simulink model "Optimized_Quadrotor_Trajectory_PID_Control"  (R2021b)
settings: Solver=ode3  StartTime=0.0  StopTime=70  FixedStep=1e-3  RelTol=1e-3
libraries: vrlib x2
(part 1 of 2)
settings Model: Creator=hellb  LastModifiedBy=hellb
settings SolverCC: AlgebraicLoopSolver=TrustRegion
settings DataIOCC: ReturnWorkspaceOutputs=off
settings DebuggingCC: SFMachineParentedDataDiag=warning  ArithmeticOperatorsInVariantConditions=warning
settings SFSimCC: SimUseLocalCustomCode=off  CustomCodeUndefinedFunction=UseInterfaceOnly
settings RTWCC: RTWUseLocalCustomCode=off

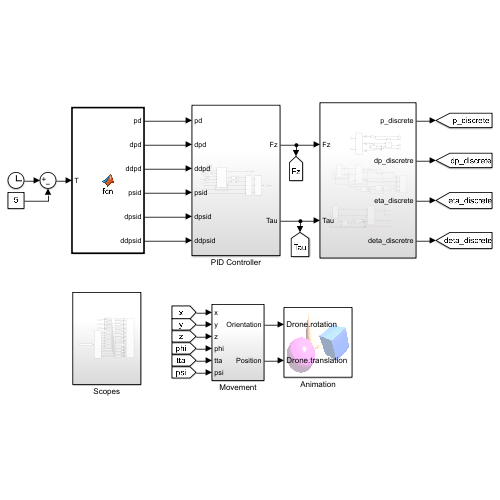
[thumbnail: Simulink's stored preview of the top-level diagram]
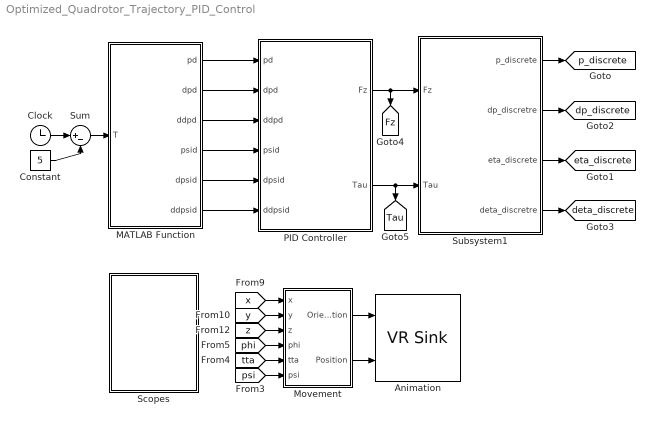
== system Optimized_Quadrotor_Trajectory_PID_Control ==
  Animation : vrlib/VR Sink  InstantiateOnLoad=on  SampleTime=0.01  ViewEnable=on  RemoteChange=off  RemoteView=off  FieldsWritten=Drone.rotation.4.1.1.double#Drone.translation.3.1.1.double  WorldFileName=Animation\hummingbird.wrl  AutoView=off  VideoDimensions=[]  AllowVariableSize=off
  Clock : Clock
  Constant : Constant  Value=5
  MATLAB Function : MATLAB Function  TreatAsAtomicUnit=on
  Movement : Subsystem
  PID Controller : Subsystem
  Scopes : Subsystem
  Subsystem1 : Subsystem
  Sum : Sum  Inputs=|+-
  tag scope: Fz=global, Tau=global, deta_discrete=global, dp_discrete=global, eta_discrete=global, p_discrete=global
  wires:
  [tta] -> Movement/5(tta)
  Movement/1(Orientation) -> Animation/1
  [z] -> Movement/3(z)
  Movement/2(Position) -> Animation/2
  [psi] -> Movement/6(psi)
  [y] -> Movement/2(y)
  [phi] -> Movement/4(phi)
  [x] -> Movement/1(x)
  Clock/1 -> Sum/1
  PID Controller/2(Tau) -> [Tau], Subsystem1/2(Tau)
  Subsystem1/1(p_discrete) -> [p_discrete]
  Subsystem1/3(eta_discrete) -> [eta_discrete]
  PID Controller/1(Fz) -> [Fz], Subsystem1/1(Fz)
  Subsystem1/2(dp_discretre) -> [dp_discrete]
  Subsystem1/4(deta_discretre) -> [deta_discrete]
  Sum/1 -> MATLAB Function/1(T)
  Constant/1 -> Sum/2
  MATLAB Function/1(pd) -> PID Controller/1(pd)
  MATLAB Function/2(dpd) -> PID Controller/2(dpd)
  MATLAB Function/3(ddpd) -> PID Controller/3(ddpd)
  MATLAB Function/4(psid) -> PID Controller/4(psid)
  MATLAB Function/5(dpsid) -> PID Controller/5(dpsid)
  MATLAB Function/6(ddpsid) -> PID Controller/6(ddpsid)

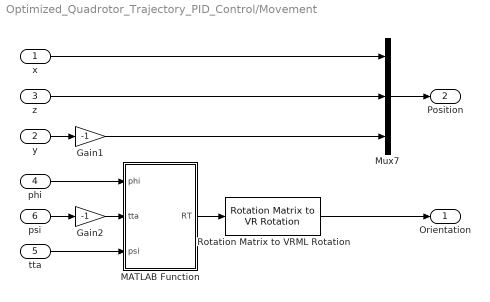
== system Optimized_Quadrotor_Trajectory_PID_Control/Movement ==
  x : Inport
  y : Inport  Port=2
  z : Inport  Port=3
  phi : Inport  Port=4
  tta : Inport  Port=5
  psi : Inport  Port=6
  Gain1 : Gain  Gain=-1
  Gain2 : Gain  Gain=-1
  MATLAB Function : MATLAB Function  TreatAsAtomicUnit=on
  Mux7 : Mux  Inputs=3
  Rotation Matrix to VRML Rotation : vrlib/Utilities/Rotation Matrix to VR Rotation  maxzero=1e-12
      settings: SourceProductBaseCode=SL
  Orientation : Outport  VectorParamsAs1DForOutWhenUnconnected=off
  Position : Outport  Port=2  VectorParamsAs1DForOutWhenUnconnected=off
  wires:
  Gain1/1 -> Mux7/3
  Rotation Matrix to VRML Rotation/1 -> Orientation/1
  Mux7/1 -> Position/1
  x/1 -> Mux7/1
  psi/1 -> Gain2/1
  MATLAB Function/1(RT) -> Rotation Matrix to VRML Rotation/1
  phi/1 -> MATLAB Function/1(phi)
  y/1 -> Gain1/1
  z/1 -> Mux7/2
  Gain2/1 -> MATLAB Function/2(tta)
  tta/1 -> MATLAB Function/3(psi)

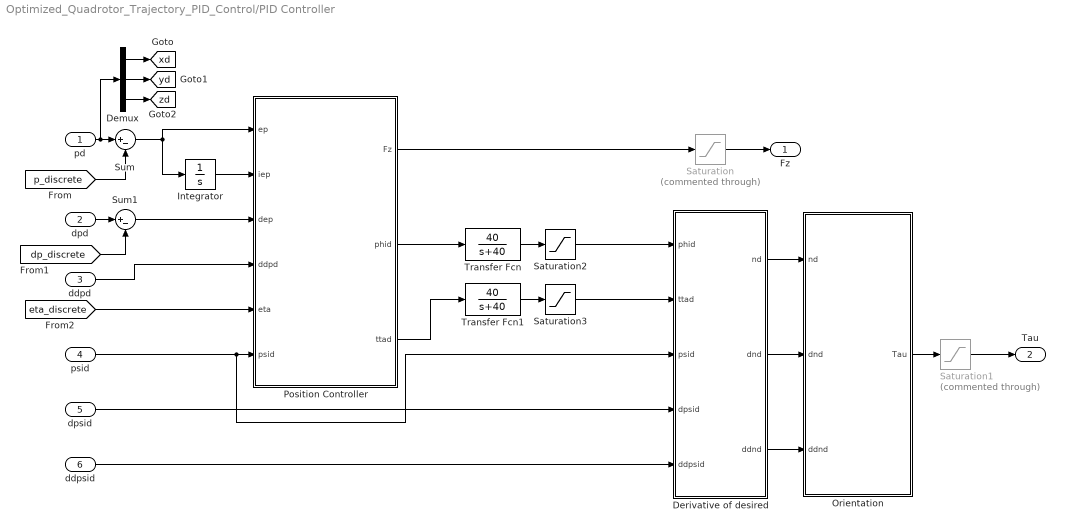
== system Optimized_Quadrotor_Trajectory_PID_Control/PID Controller ==
  pd : Inport
  dpd : Inport  Port=2
  ddpd : Inport  Port=3
  psid : Inport  Port=4
  dpsid : Inport  Port=5
  ddpsid : Inport  Port=6
  Demux : Demux  Outputs=3
  Derivative of desired : Subsystem
  Integrator : Integrator  InitialCondition=[0;0;0]
  Orientation : Subsystem
  Position Controller : MATLAB Function  TreatAsAtomicUnit=on
  Saturation : Saturate  Commented=through  UpperLimit=25  LowerLimit=0
  Saturation1 : Saturate  Commented=through  UpperLimit=0.2*(25/4)  LowerLimit=-0.2*(25/4)
  Saturation2 : Saturate  UpperLimit=0.25  LowerLimit=-0.25
  Saturation3 : Saturate  UpperLimit=0.25  LowerLimit=-0.25
  Sum : Sum  Inputs=|+-
  Sum1 : Sum  Inputs=|+-
  Transfer Fcn : TransferFcn  Numerator=[40]  Denominator=[1 40]
  Transfer Fcn1 : TransferFcn  Numerator=[40]  Denominator=[1 40]
  Fz : Outport  VectorParamsAs1DForOutWhenUnconnected=off
  Tau : Outport  Port=2  VectorParamsAs1DForOutWhenUnconnected=off
  tag scope: xd=global, yd=global, zd=global
  wires:
  ddpd/1 -> Position Controller/4(ddpd)
  dpd/1 -> Sum1/1
  [dp_discrete] -> Sum1/2
  Integrator/1 -> Position Controller/2(iep)
  [eta_discrete] -> Position Controller/5(eta)
  Derivative of desired/1(nd) -> Orientation/1(nd)
  Derivative of desired/2(dnd) -> Orientation/2(dnd)
  pd/1 -> Demux/1, Sum/1
  [p_discrete] -> Sum/2
  Sum/1 -> Integrator/1, Position Controller/1(ep)
  Sum1/1 -> Position Controller/3(dep)
  Demux/1 -> [xd]
  Demux/3 -> [zd]
  Demux/2 -> [yd]
  psid/1 -> Derivative of desired/3(psid), Position Controller/6(psid)
  Position Controller/3(ttad) -> Transfer Fcn1/1
  Position Controller/1(Fz) -> Saturation/1
  Orientation/1(Tau) -> Saturation1/1
  Saturation/1 -> Fz/1
  Saturation1/1 -> Tau/1
  dpsid/1 -> Derivative of desired/4(dpsid)
  ddpsid/1 -> Derivative of desired/5(ddpsid)
  Derivative of desired/3(ddnd) -> Orientation/3(ddnd)
  Position Controller/2(phid) -> Transfer Fcn/1
  Saturation2/1 -> Derivative of desired/1(phid)
  Transfer Fcn/1 -> Saturation2/1
  Transfer Fcn1/1 -> Saturation3/1
  Saturation3/1 -> Derivative of desired/2(ttad)

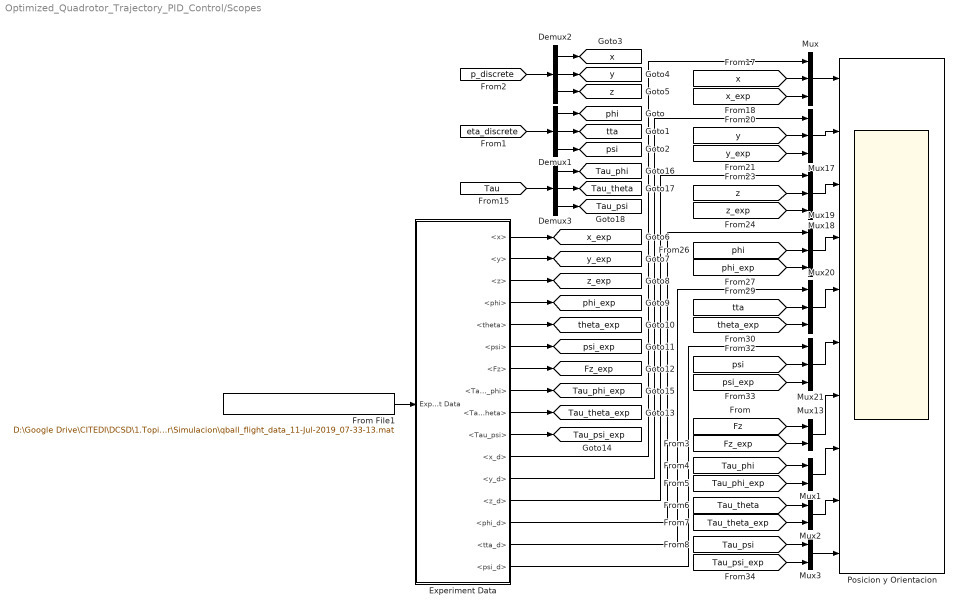
== system Optimized_Quadrotor_Trajectory_PID_Control/Scopes ==
  Demux1 : Demux  Outputs=3
  Demux2 : Demux  Outputs=3
  Demux3 : Demux  Outputs=3
  Experiment Data : Subsystem
  From File1 : FromFile  FileName=D:\Google Drive\CITEDI\DCSD\1.Topicos de Identificacion y Control Adaptable\Optimizacion Quadrotor\Simulacion\qball_flight_data_11-Jul-2019_07-33-13.mat  SampleTime=0
  Mux{,17..21} (6 alike) : Mux  Inputs=3
  Mux{1..3,13} (4 alike) : Mux  Inputs=2
  Posicion y Orientacion : Scope  NumInputPorts=10
  tag scope: Fz_exp=global, Tau_phi=global, Tau_phi_exp=global, Tau_psi=global, Tau_psi_exp=global, Tau_theta=global, Tau_theta_exp=global, phi=global, phi_exp=global, psi=global, psi_exp=global, theta_exp=global, tta=global, x=global, x_exp=global, y=global, y_exp=global, z=global, z_exp=global
  wires:
  Demux1/3 -> [psi]
  Demux1/2 -> [tta]
  [eta_discrete] -> Demux1/1
  Demux1/1 -> [phi]
  Demux2/1 -> [x]
  [p_discrete] -> Demux2/1
  Demux2/2 -> [y]
  Demux2/3 -> [z]
  [Fz] -> Mux13/1
  [Tau] -> Demux3/1
  Mux/1 -> Posicion y Orientacion/1
  [x] -> Mux/2
  [x_exp] -> Mux/3
  [y_exp] -> Mux17/3
  [y] -> Mux17/2
  Mux17/1 -> Posicion y Orientacion/2
  Mux18/1 -> Posicion y Orientacion/3
  [z] -> Mux18/2
  [z_exp] -> Mux18/3
  [phi_exp] -> Mux19/3
  [phi] -> Mux19/2
  Mux19/1 -> Posicion y Orientacion/4
  Mux20/1 -> Posicion y Orientacion/5
  [tta] -> Mux20/2
  [theta_exp] -> Mux20/3
  [psi_exp] -> Mux21/3
  [psi] -> Mux21/2
  Mux21/1 -> Posicion y Orientacion/6
  From File1/1 -> Experiment Data/1(Experiment Data)
  Experiment Data/1(<x>) -> [x_exp]
  Experiment Data/2(<y>) -> [y_exp]
  Experiment Data/3(<z>) -> [z_exp]
  Experiment Data/4(<phi>) -> [phi_exp]
  Experiment Data/5(<theta>) -> [theta_exp]
  Experiment Data/6(<psi>) -> [psi_exp]
  Experiment Data/7(<Fz>) -> [Fz_exp]
  Experiment Data/8(<Tau_phi>) -> [Tau_phi_exp]
  Experiment Data/9(<Tau_theta>) -> [Tau_theta_exp]
  Experiment Data/10(<Tau_psi>) -> [Tau_psi_exp]
  [Fz_exp] -> Mux13/2
  Demux3/1 -> [Tau_phi]
  Demux3/2 -> [Tau_theta]
  Demux3/3 -> [Tau_psi]
  [Tau_phi] -> Mux1/1
  [Tau_theta] -> Mux2/1
  [Tau_psi] -> Mux3/1
  Experiment Data/11(<x_d>) -> Mux/1
  Experiment Data/12(<y_d>) -> Mux17/1
  Experiment Data/13(<z_d>) -> Mux18/1
  Experiment Data/16(<psi_d>) -> Mux21/1
  Experiment Data/14(<phi_d>) -> Mux19/1
  Experiment Data/15(<tta_d>) -> Mux20/1
  Mux13/1 -> Posicion y Orientacion/7
  Mux1/1 -> Posicion y Orientacion/8
  Mux2/1 -> Posicion y Orientacion/9
  Mux3/1 -> Posicion y Orientacion/10
  [Tau_phi_exp] -> Mux1/2
  [Tau_theta_exp] -> Mux2/2
  [Tau_psi_exp] -> Mux3/2

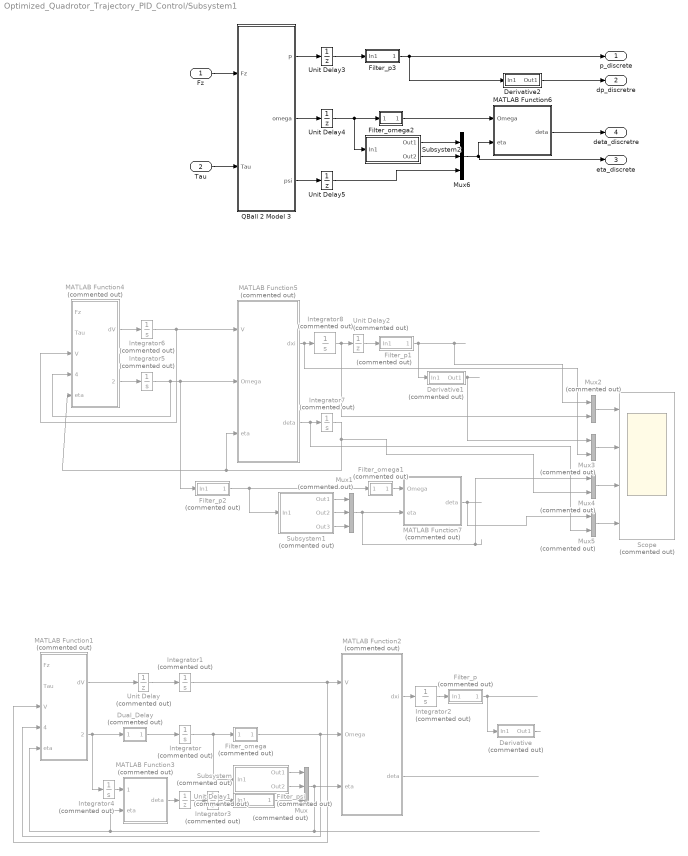
== system Optimized_Quadrotor_Trajectory_PID_Control/Subsystem1 ==
  Fz : Inport
  Tau : Inport  Port=2
  Derivative : Subsystem  Commented=on
  Derivative1 : Subsystem  Commented=on
  Derivative2 : Subsystem
  Dual_Delay : Subsystem  Commented=on
  Filter_omega : Subsystem  Commented=on
  Filter_omega1 : Subsystem  Commented=on
  Filter_omega2 : Subsystem
  Filter_p : Subsystem  Commented=on
  Filter_p1 : Subsystem  Commented=on
  Filter_p2 : Subsystem  Commented=on
  Filter_p3 : Subsystem
  Filter_psi : Subsystem  Commented=on
  Integrator{,1,3..7} (7 alike) : Integrator  Commented=on  InitialCondition=[0;0;0]
  Integrator2 : Integrator  Commented=on  InitialCondition=[0;0;0.3]  LimitOutput=on  LowerSaturationLimit=[-inf;-inf;0.3]
  Integrator8 : Integrator  Commented=on  InitialCondition=[0;0;0.3]  LimitOutput=on  LowerSaturationLimit=[-inf;-inf;0.3]
  MATLAB Function1 : MATLAB Function  Commented=on  TreatAsAtomicUnit=on
  MATLAB Function2 : MATLAB Function  Commented=on  TreatAsAtomicUnit=on
  MATLAB Function3 : MATLAB Function  Commented=on  TreatAsAtomicUnit=on
  MATLAB Function4 : MATLAB Function  Commented=on  TreatAsAtomicUnit=on
  MATLAB Function5 : MATLAB Function  Commented=on  TreatAsAtomicUnit=on
  MATLAB Function6 : MATLAB Function  TreatAsAtomicUnit=on
  MATLAB Function7 : MATLAB Function  Commented=on  TreatAsAtomicUnit=on
  Mux : Mux  Commented=on  Inputs=3
  Mux1 : Mux  Commented=on  Inputs=3
  Mux{2..5} (4 alike) : Mux  Commented=on  Inputs=2
  Mux6 : Mux  Inputs=3
  QBall 2 Model 3 : Subsystem
  Scope : Scope  Commented=on  NumInputPorts=4
  Subsystem : Subsystem  Commented=on
  Subsystem1 : Subsystem  Commented=on
  Subsystem2 : Subsystem
  Unit Delay : UnitDelay  Commented=on  SampleTime=0.033  HasFrameUpgradeWarning=on
  Unit Delay1 : UnitDelay  Commented=on  SampleTime=0.033  HasFrameUpgradeWarning=on
  Unit Delay2 : UnitDelay  Commented=on  SampleTime=0.033  HasFrameUpgradeWarning=on
  Unit Delay3 : UnitDelay  InitialCondition=[0;0;0.3]  SampleTime=0.033  HasFrameUpgradeWarning=on
  Unit Delay4 : UnitDelay  InitialCondition=[0;0;0]  SampleTime=0.002  HasFrameUpgradeWarning=on
  Unit Delay5 : UnitDelay  SampleTime=0.033  HasFrameUpgradeWarning=on
  p_discrete : Outport  VectorParamsAs1DForOutWhenUnconnected=off
  dp_discretre : Outport  Port=2  VectorParamsAs1DForOutWhenUnconnected=off
  eta_discrete : Outport  Port=3  VectorParamsAs1DForOutWhenUnconnected=off
  deta_discretre : Outport  Port=4  VectorParamsAs1DForOutWhenUnconnected=off
  wires:
  MATLAB Function1/1(dV) -> Unit Delay/1
  Fz/1 -> QBall 2 Model 3/1(Fz)
  MATLAB Function1/2(dOmega) -> Dual_Delay/1(In), Integrator4/1
  Integrator2/1 -> Filter_p/1(In1)
  Tau/1 -> QBall 2 Model 3/2(Tau)
  Integrator1/1 -> MATLAB Function2/1(V), MATLAB Function1/3(V)
  Filter_p/1(Out1) -> Derivative/1(In1)
  Filter_omega/1(Out) -> MATLAB Function2/2(Omega), MATLAB Function1/4(Omega)
  Filter_psi/1(psi_discrete) -> Mux/3
  Integrator/1 -> Filter_omega/1(In), Subsystem/1(In1)
  Subsystem/1(Out1) -> Mux/1
  Subsystem/2(Out2) -> Mux/2
  Unit Delay/1 -> Integrator1/1
  Dual_Delay/1(Out) -> Integrator/1
  MATLAB Function2/2(deta) -> ?
  MATLAB Function2/1(dxi) -> Integrator2/1
  Derivative/1(Out1) -> ?
  Integrator4/1 -> MATLAB Function3/1(Omega)
  Mux/1 -> MATLAB Function2/3(eta), MATLAB Function3/2(eta), MATLAB Function1/5(eta)
  MATLAB Function3/1(deta) -> Unit Delay1/1
  Unit Delay1/1 -> Integrator3/1
  Integrator3/1 -> Filter_psi/1(In1)
  MATLAB Function4/1(dV) -> Integrator6/1
  Integrator6/1 -> MATLAB Function5/1(V), MATLAB Function4/3(V)
  MATLAB Function5/2(deta) -> Mux5/2, Integrator7/1
  Integrator7/1 -> Mux4/2, MATLAB Function4/5(eta), MATLAB Function5/3(eta)
  Derivative1/1(Out1) -> Mux3/1
  Filter_p1/1(Out1) -> Mux2/1, Derivative1/1(In1)
  Integrator8/1 -> Mux2/2, Unit Delay2/1
  MATLAB Function5/1(dxi) -> Mux3/2, Integrator8/1
  Unit Delay2/1 -> Filter_p1/1(In1)
  Subsystem1/1(Out1) -> Mux1/1
  MATLAB Function4/2(dOmega) -> Integrator5/1
  Mux1/1 -> Mux4/1, MATLAB Function7/2(eta)
  Subsystem1/2(Out2) -> Mux1/2
  Integrator5/1 -> MATLAB Function4/4(Omega), Filter_p2/1(In1), MATLAB Function5/2(Omega)
  Filter_omega1/1(Out) -> MATLAB Function7/1(Omega)
  MATLAB Function7/1(deta) -> Mux5/1
  Mux2/1 -> Scope/1
  Mux3/1 -> Scope/2
  Mux4/1 -> Scope/3
  Mux5/1 -> Scope/4
  Filter_p2/1(Out1) -> Subsystem1/1(In1), Filter_omega1/1(In)
  Subsystem1/3(Out3) -> Mux1/3
  Unit Delay3/1 -> Filter_p3/1(In1)
  Filter_p3/1(Out1) -> p_discrete/1, Derivative2/1(In1)
  QBall 2 Model 3/1(p) -> Unit Delay3/1
  Derivative2/1(Out1) -> dp_discretre/1
  QBall 2 Model 3/2(omega) -> Unit Delay4/1
  QBall 2 Model 3/3(psi) -> Unit Delay5/1
  Unit Delay4/1 -> Subsystem2/1(In1), Filter_omega2/1(In)
  Filter_omega2/1(Out) -> MATLAB Function6/1(Omega)
  MATLAB Function6/1(deta) -> deta_discretre/1
  Subsystem2/1(Out1) -> Mux6/1
  Subsystem2/2(Out2) -> Mux6/2
  Unit Delay5/1 -> Mux6/3
  Mux6/1 -> MATLAB Function6/2(eta), eta_discrete/1

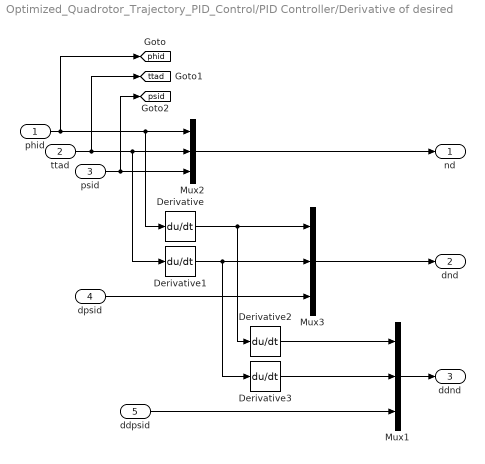
== system Optimized_Quadrotor_Trajectory_PID_Control/PID Controller/Derivative of desired ==
  phid : Inport
  ttad : Inport  Port=2
  psid : Inport  Port=3
  dpsid : Inport  Port=4
  ddpsid : Inport  Port=5
  Derivative{,1..3} (4 alike) : Derivative
  Mux1 : Mux  Inputs=3
  Mux2 : Mux  Inputs=3
  Mux3 : Mux  Inputs=3
  nd : Outport  VectorParamsAs1DForOutWhenUnconnected=off
  dnd : Outport  Port=2  VectorParamsAs1DForOutWhenUnconnected=off
  ddnd : Outport  Port=3  VectorParamsAs1DForOutWhenUnconnected=off
  tag scope: phid=global, psid=global, ttad=global
  wires:
  ttad/1 -> [ttad], Derivative1/1, Mux2/2
  Derivative/1 -> Derivative2/1, Mux3/1
  phid/1 -> [phid], Derivative/1, Mux2/1
  Mux3/1 -> dnd/1
  Derivative1/1 -> Derivative3/1, Mux3/2
  Mux2/1 -> nd/1
  psid/1 -> [psid], Mux2/3
  dpsid/1 -> Mux3/3
  ddpsid/1 -> Mux1/3
  Derivative3/1 -> Mux1/2
  Mux1/1 -> ddnd/1
  Derivative2/1 -> Mux1/1

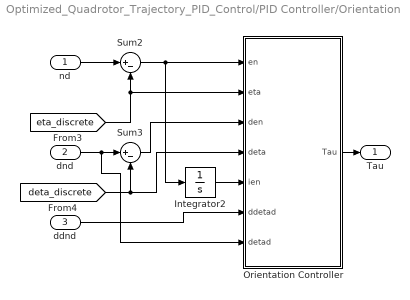
== system Optimized_Quadrotor_Trajectory_PID_Control/PID Controller/Orientation ==
  nd : Inport
  dnd : Inport  Port=2
  ddnd : Inport  Port=3
  Integrator2 : Integrator  InitialCondition=[0;0;0]
  Orientation Controller : MATLAB Function  TreatAsAtomicUnit=on
  Sum2 : Sum  Inputs=|+-
  Sum3 : Sum  Inputs=|+-
  Tau : Outport  VectorParamsAs1DForOutWhenUnconnected=off
  wires:
  [deta_discrete] -> Orientation Controller/4(deta), Sum3/2
  [eta_discrete] -> Sum2/2, Orientation Controller/2(eta)
  dnd/1 -> Orientation Controller/7(detad), Sum3/1
  Orientation Controller/1(Tau) -> Tau/1
  Sum2/1 -> Integrator2/1, Orientation Controller/1(en)
  Sum3/1 -> Orientation Controller/3(den)
  nd/1 -> Sum2/1
  Integrator2/1 -> Orientation Controller/5(ien)
  ddnd/1 -> Orientation Controller/6(ddetad)

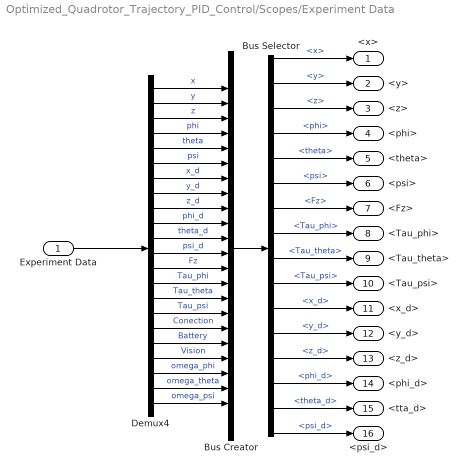
== system Optimized_Quadrotor_Trajectory_PID_Control/Scopes/Experiment Data ==
  Experiment Data : Inport
  Bus Creator : BusCreator  Inputs=22
  Bus Selector : BusSelector  OutputSignals=x,y,z,phi,theta,psi,Fz,Tau_phi,Tau_theta,Tau_psi,x_d,y_d,z_d,phi_d,theta_d,psi_d
  Demux4 : Demux  Outputs=22
  <x> : Outport  VectorParamsAs1DForOutWhenUnconnected=off
  <y> : Outport  Port=2  VectorParamsAs1DForOutWhenUnconnected=off
  <z> : Outport  Port=3  VectorParamsAs1DForOutWhenUnconnected=off
  <phi> : Outport  Port=4  VectorParamsAs1DForOutWhenUnconnected=off
  <theta> : Outport  Port=5  VectorParamsAs1DForOutWhenUnconnected=off
  <psi> : Outport  Port=6  VectorParamsAs1DForOutWhenUnconnected=off
  <Fz> : Outport  Port=7  VectorParamsAs1DForOutWhenUnconnected=off
  <Tau_phi> : Outport  Port=8  VectorParamsAs1DForOutWhenUnconnected=off
  <Tau_theta> : Outport  Port=9  VectorParamsAs1DForOutWhenUnconnected=off
  <Tau_psi> : Outport  Port=10  VectorParamsAs1DForOutWhenUnconnected=off
  <x_d> : Outport  Port=11  VectorParamsAs1DForOutWhenUnconnected=off
  <y_d> : Outport  Port=12  VectorParamsAs1DForOutWhenUnconnected=off
  <z_d> : Outport  Port=13  VectorParamsAs1DForOutWhenUnconnected=off
  <phi_d> : Outport  Port=14  VectorParamsAs1DForOutWhenUnconnected=off
  <tta_d> : Outport  Port=15  VectorParamsAs1DForOutWhenUnconnected=off
  <psi_d> : Outport  Port=16  VectorParamsAs1DForOutWhenUnconnected=off
  wires:
  Demux4/3 -> Bus Creator/3  "z"
  Demux4/22 -> Bus Creator/22  "omega_psi"
  Demux4/18 -> Bus Creator/18  "Battery"
  Demux4/15 -> Bus Creator/15  "Tau_theta"
  Demux4/6 -> Bus Creator/6  "psi"
  Demux4/13 -> Bus Creator/13  "Fz"
  Demux4/10 -> Bus Creator/10  "phi_d"
  Demux4/9 -> Bus Creator/9  "z_d"
  Demux4/5 -> Bus Creator/5  "theta"
  Demux4/14 -> Bus Creator/14  "Tau_phi"
  Demux4/11 -> Bus Creator/11  "theta_d"
  Demux4/2 -> Bus Creator/2  "y"
  Demux4/19 -> Bus Creator/19  "Vision"
  Bus Selector/6 -> <psi>/1  "<psi>"
  Bus Selector/9 -> <Tau_theta>/1  "<Tau_theta>"
  Bus Selector/5 -> <theta>/1  "<theta>"
  Demux4/4 -> Bus Creator/4  "phi"
  Demux4/17 -> Bus Creator/17  "Conection"
  Bus Creator/1 -> Bus Selector/1
  Demux4/16 -> Bus Creator/16  "Tau_psi"
  Demux4/20 -> Bus Creator/20  "omega_phi"
  Demux4/12 -> Bus Creator/12  "psi_d"
  Demux4/1 -> Bus Creator/1  "x"
  Demux4/7 -> Bus Creator/7  "x_d"
  Demux4/21 -> Bus Creator/21  "omega_theta"
  Bus Selector/8 -> <Tau_phi>/1  "<Tau_phi>"
  Demux4/8 -> Bus Creator/8  "y_d"
  Bus Selector/2 -> <y>/1  "<y>"
  Bus Selector/3 -> <z>/1  "<z>"
  Bus Selector/1 -> <x>/1  "<x>"
  Bus Selector/7 -> <Fz>/1  "<Fz>"
  Bus Selector/4 -> <phi>/1  "<phi>"
  Bus Selector/10 -> <Tau_psi>/1  "<Tau_psi>"
  Experiment Data/1 -> Demux4/1
  Bus Selector/11 -> <x_d>/1  "<x_d>"
  Bus Selector/12 -> <y_d>/1  "<y_d>"
  Bus Selector/13 -> <z_d>/1  "<z_d>"
  Bus Selector/16 -> <psi_d>/1  "<psi_d>"
  Bus Selector/15 -> <tta_d>/1  "<theta_d>"
  Bus Selector/14 -> <phi_d>/1  "<phi_d>"

== system Optimized_Quadrotor_Trajectory_PID_Control/Subsystem1/Derivative ==
  In1 : Inport
  Demux3 : Demux  Outputs=3
  Mux1 : Mux  Inputs=3
  Subsystem : Subsystem
  Transfer Fcn : TransferFcn  Numerator=[20 0]  Denominator=[1 20]
  Transfer Fcn1 : TransferFcn  Numerator=[20 0]  Denominator=[1 20]
  Transfer Fcn2 : TransferFcn  Numerator=[10 0]  Denominator=[1 10]
  Out1 : Outport  VectorParamsAs1DForOutWhenUnconnected=off
  wires:
  Mux1/1 -> Out1/1
  Transfer Fcn2/1 -> Subsystem/1(In1)
  Demux3/3 -> Transfer Fcn2/1
  Demux3/1 -> Transfer Fcn/1
  Demux3/2 -> Transfer Fcn1/1
  In1/1 -> Demux3/1
  Transfer Fcn/1 -> Mux1/1
  Transfer Fcn1/1 -> Mux1/2
  Subsystem/1(Out1) -> Mux1/3

== system Optimized_Quadrotor_Trajectory_PID_Control/Subsystem1/Derivative1 ==
  In1 : Inport
  Demux3 : Demux  Outputs=3
  Mux1 : Mux  Inputs=3
  Subsystem : Subsystem
  Transfer Fcn : TransferFcn  Numerator=[20 0]  Denominator=[1 20]
  Transfer Fcn1 : TransferFcn  Numerator=[20 0]  Denominator=[1 20]
  Transfer Fcn2 : TransferFcn  Numerator=[10 0]  Denominator=[1 10]
  Out1 : Outport  VectorParamsAs1DForOutWhenUnconnected=off
  wires:
  Mux1/1 -> Out1/1
  Transfer Fcn2/1 -> Subsystem/1(In1)
  Demux3/3 -> Transfer Fcn2/1
  Demux3/1 -> Transfer Fcn/1
  Demux3/2 -> Transfer Fcn1/1
  In1/1 -> Demux3/1
  Transfer Fcn/1 -> Mux1/1
  Transfer Fcn1/1 -> Mux1/2
  Subsystem/1(Out1) -> Mux1/3

== system Optimized_Quadrotor_Trajectory_PID_Control/Subsystem1/Derivative2 ==
  In1 : Inport
  Demux3 : Demux  Outputs=3
  Mux1 : Mux  Inputs=3
  Subsystem : Subsystem
  Transfer Fcn : TransferFcn  Numerator=[20 0]  Denominator=[1 20]
  Transfer Fcn1 : TransferFcn  Numerator=[20 0]  Denominator=[1 20]
  Transfer Fcn2 : TransferFcn  Numerator=[10 0]  Denominator=[1 10]
  Out1 : Outport  VectorParamsAs1DForOutWhenUnconnected=off
  wires:
  Subsystem/1(Out1) -> Mux1/3
  Transfer Fcn1/1 -> Mux1/2
  Transfer Fcn/1 -> Mux1/1
  In1/1 -> Demux3/1
  Demux3/2 -> Transfer Fcn1/1
  Demux3/1 -> Transfer Fcn/1
  Demux3/3 -> Transfer Fcn2/1
  Transfer Fcn2/1 -> Subsystem/1(In1)
  Mux1/1 -> Out1/1

== system Optimized_Quadrotor_Trajectory_PID_Control/Subsystem1/Dual_Delay ==
  In : Inport
  Demux3 : Demux  Outputs=3
  Mux1 : Mux  Inputs=3
  Unit Delay : UnitDelay  SampleTime=0.002  HasFrameUpgradeWarning=on
  Unit Delay1 : UnitDelay  SampleTime=0.002  HasFrameUpgradeWarning=on
  Unit Delay2 : UnitDelay  SampleTime=0.033  HasFrameUpgradeWarning=on
  Out : Outport  VectorParamsAs1DForOutWhenUnconnected=off
  wires:
  Demux3/3 -> Unit Delay2/1
  Demux3/2 -> Unit Delay1/1
  Demux3/1 -> Unit Delay/1
  Unit Delay2/1 -> Mux1/3
  Unit Delay1/1 -> Mux1/2
  Unit Delay/1 -> Mux1/1
  In/1 -> Demux3/1
  Mux1/1 -> Out/1

== system Optimized_Quadrotor_Trajectory_PID_Control/Subsystem1/Filter_omega ==
  In : Inport
  Demux3 : Demux  Outputs=3
  Mux1 : Mux  Inputs=3
  Transfer Fcn : TransferFcn  Numerator=[40]  Denominator=[1 40]
  Transfer Fcn1 : TransferFcn  Numerator=[40]  Denominator=[1 40]
  Transfer Fcn2 : TransferFcn  Numerator=[40]  Denominator=[1 40]
  Out : Outport  VectorParamsAs1DForOutWhenUnconnected=off
  wires:
  Demux3/3 -> Transfer Fcn2/1
  Demux3/2 -> Transfer Fcn1/1
  Demux3/1 -> Transfer Fcn/1
  Transfer Fcn2/1 -> Mux1/3
  Transfer Fcn1/1 -> Mux1/2
  Transfer Fcn/1 -> Mux1/1
  In/1 -> Demux3/1
  Mux1/1 -> Out/1

== system Optimized_Quadrotor_Trajectory_PID_Control/Subsystem1/Filter_omega1 ==
  In : Inport
  Demux3 : Demux  Outputs=3
  Mux1 : Mux  Inputs=3
  Transfer Fcn : TransferFcn  Numerator=[40]  Denominator=[1 40]
  Transfer Fcn1 : TransferFcn  Numerator=[40]  Denominator=[1 40]
  Transfer Fcn2 : TransferFcn  Numerator=[40]  Denominator=[1 40]
  Out : Outport  VectorParamsAs1DForOutWhenUnconnected=off
  wires:
  Mux1/1 -> Out/1
  In/1 -> Demux3/1
  Transfer Fcn/1 -> Mux1/1
  Transfer Fcn1/1 -> Mux1/2
  Transfer Fcn2/1 -> Mux1/3
  Demux3/1 -> Transfer Fcn/1
  Demux3/2 -> Transfer Fcn1/1
  Demux3/3 -> Transfer Fcn2/1

== system Optimized_Quadrotor_Trajectory_PID_Control/Subsystem1/Filter_omega2 ==
  In : Inport
  Demux3 : Demux  Outputs=3
  Mux1 : Mux  Inputs=3
  Transfer Fcn : TransferFcn  Numerator=[40]  Denominator=[1 40]
  Transfer Fcn1 : TransferFcn  Numerator=[40]  Denominator=[1 40]
  Transfer Fcn2 : TransferFcn  Numerator=[40]  Denominator=[1 40]
  Out : Outport  VectorParamsAs1DForOutWhenUnconnected=off
  wires:
  Demux3/3 -> Transfer Fcn2/1
  Demux3/2 -> Transfer Fcn1/1
  Demux3/1 -> Transfer Fcn/1
  Transfer Fcn2/1 -> Mux1/3
  Transfer Fcn1/1 -> Mux1/2
  Transfer Fcn/1 -> Mux1/1
  In/1 -> Demux3/1
  Mux1/1 -> Out/1

== system Optimized_Quadrotor_Trajectory_PID_Control/Subsystem1/Filter_p ==
  In1 : Inport
  Demux3 : Demux  Outputs=3
  Mux1 : Mux  Inputs=3
  Transfer Fcn : TransferFcn  Numerator=[50]  Denominator=[1 50]
  Transfer Fcn1 : TransferFcn  Numerator=[50]  Denominator=[1 50]
  Transfer Fcn2 : TransferFcn  Numerator=[50]  Denominator=[1 50]
  Out1 : Outport  VectorParamsAs1DForOutWhenUnconnected=off
  wires:
  In1/1 -> Demux3/1
  Mux1/1 -> Out1/1
  Transfer Fcn/1 -> Mux1/3
  Transfer Fcn1/1 -> Mux1/2
  Transfer Fcn2/1 -> Mux1/1
  Demux3/1 -> Transfer Fcn2/1
  Demux3/2 -> Transfer Fcn1/1
  Demux3/3 -> Transfer Fcn/1

== system Optimized_Quadrotor_Trajectory_PID_Control/Subsystem1/Filter_p1 ==
  In1 : Inport
  Demux3 : Demux  Outputs=3
  Mux1 : Mux  Inputs=3
  Transfer Fcn : TransferFcn  Numerator=[50]  Denominator=[1 50]
  Transfer Fcn1 : TransferFcn  Numerator=[50]  Denominator=[1 50]
  Transfer Fcn2 : TransferFcn  Numerator=[50]  Denominator=[1 50]
  Out1 : Outport  VectorParamsAs1DForOutWhenUnconnected=off
  wires:
  In1/1 -> Demux3/1
  Mux1/1 -> Out1/1
  Transfer Fcn/1 -> Mux1/3
  Transfer Fcn1/1 -> Mux1/2
  Transfer Fcn2/1 -> Mux1/1
  Demux3/1 -> Transfer Fcn2/1
  Demux3/2 -> Transfer Fcn1/1
  Demux3/3 -> Transfer Fcn/1

== system Optimized_Quadrotor_Trajectory_PID_Control/Subsystem1/Filter_p2 ==
  In1 : Inport
  Demux3 : Demux  Outputs=3
  Mux1 : Mux  Inputs=3
  Unit Delay : UnitDelay  SampleTime=0.002  HasFrameUpgradeWarning=on
  Unit Delay1 : UnitDelay  SampleTime=0.002  HasFrameUpgradeWarning=on
  Unit Delay2 : UnitDelay  SampleTime=0.033  HasFrameUpgradeWarning=on
  Out1 : Outport  VectorParamsAs1DForOutWhenUnconnected=off
  wires:
  Demux3/3 -> Unit Delay2/1
  Demux3/2 -> Unit Delay1/1
  Demux3/1 -> Unit Delay/1
  Mux1/1 -> Out1/1
  In1/1 -> Demux3/1
  Unit Delay/1 -> Mux1/1
  Unit Delay1/1 -> Mux1/2
  Unit Delay2/1 -> Mux1/3

== system Optimized_Quadrotor_Trajectory_PID_Control/Subsystem1/Filter_p3 ==
  In1 : Inport
  Demux3 : Demux  Outputs=3
  Mux1 : Mux  Inputs=3
  Transfer Fcn : TransferFcn  Numerator=[50]  Denominator=[1 50]
  Transfer Fcn1 : TransferFcn  Numerator=[50]  Denominator=[1 50]
  Transfer Fcn2 : TransferFcn  Numerator=[50]  Denominator=[1 50]
  Out1 : Outport  VectorParamsAs1DForOutWhenUnconnected=off
  wires:
  Demux3/3 -> Transfer Fcn/1
  Demux3/2 -> Transfer Fcn1/1
  Demux3/1 -> Transfer Fcn2/1
  Transfer Fcn2/1 -> Mux1/1
  Transfer Fcn1/1 -> Mux1/2
  Transfer Fcn/1 -> Mux1/3
  Mux1/1 -> Out1/1
  In1/1 -> Demux3/1

== system Optimized_Quadrotor_Trajectory_PID_Control/Subsystem1/Filter_psi ==
  In1 : Inport
  Demux3 : Demux  Outputs=3
  Terminator : Terminator
  Terminator1 : Terminator
  Transfer Fcn : TransferFcn  Numerator=[40]  Denominator=[1 40]
  Transfer Fcn1 : TransferFcn  Numerator=[40]  Denominator=[1 40]
  Transfer Fcn2 : TransferFcn  Numerator=[40]  Denominator=[1 40]
  psi_discrete : Outport  VectorParamsAs1DForOutWhenUnconnected=off
  wires:
  In1/1 -> Demux3/1
  Transfer Fcn2/1 -> psi_discrete/1
  Transfer Fcn/1 -> Terminator/1
  Transfer Fcn1/1 -> Terminator1/1
  Demux3/1 -> Transfer Fcn/1
  Demux3/2 -> Transfer Fcn1/1
  Demux3/3 -> Transfer Fcn2/1

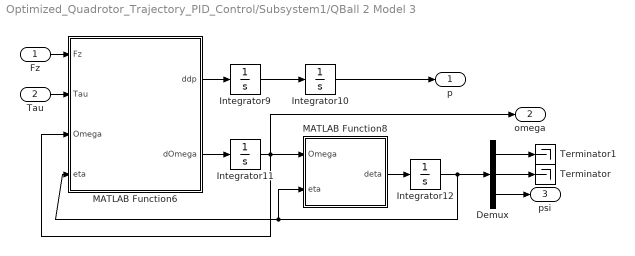
== system Optimized_Quadrotor_Trajectory_PID_Control/Subsystem1/QBall 2 Model 3 ==
  Fz : Inport
  Tau : Inport  Port=2
  Demux : Demux  Outputs=3
  Integrator10 : Integrator  InitialCondition=[0;0;0.3]  LimitOutput=on  LowerSaturationLimit=[-inf;-inf;0.3]
  Integrator11 : Integrator  InitialCondition=[0;0;0]
  Integrator12 : Integrator  InitialCondition=[0;0;0]
  Integrator9 : Integrator  InitialCondition=[0;0;0]
  MATLAB Function6 : MATLAB Function  TreatAsAtomicUnit=on
  MATLAB Function8 : MATLAB Function  TreatAsAtomicUnit=on
  Terminator : Terminator
  Terminator1 : Terminator
  p : Outport  VectorParamsAs1DForOutWhenUnconnected=off
  omega : Outport  Port=2  VectorParamsAs1DForOutWhenUnconnected=off
  psi : Outport  Port=3  VectorParamsAs1DForOutWhenUnconnected=off
  wires:
  Fz/1 -> MATLAB Function6/1(Fz)
  Integrator9/1 -> Integrator10/1
  Integrator10/1 -> p/1
  Integrator11/1 -> omega/1, MATLAB Function8/1(Omega), MATLAB Function6/3(Omega)
  Integrator12/1 -> MATLAB Function8/2(eta), MATLAB Function6/4(eta), Demux/1
  MATLAB Function6/2(dOmega) -> Integrator11/1
  Tau/1 -> MATLAB Function6/2(Tau)
  MATLAB Function6/1(ddp) -> Integrator9/1
  MATLAB Function8/1(deta) -> Integrator12/1
  Demux/3 -> psi/1
  Demux/2 -> Terminator/1
  Demux/1 -> Terminator1/1

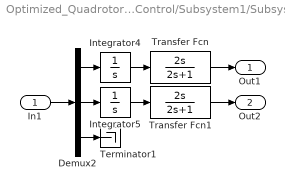
== system Optimized_Quadrotor_Trajectory_PID_Control/Subsystem1/Subsystem ==
  In1 : Inport
  Demux2 : Demux  Outputs=3
  Integrator4 : Integrator
  Integrator5 : Integrator
  Terminator1 : Terminator
  Transfer Fcn : TransferFcn  Numerator=[2 0]  Denominator=[2 1]
  Transfer Fcn1 : TransferFcn  Numerator=[2 0]  Denominator=[2 1]
  Out1 : Outport  VectorParamsAs1DForOutWhenUnconnected=off
  Out2 : Outport  Port=2  VectorParamsAs1DForOutWhenUnconnected=off
  wires:
  Transfer Fcn/1 -> Out1/1
  Integrator4/1 -> Transfer Fcn/1
  Integrator5/1 -> Transfer Fcn1/1
  Demux2/3 -> Terminator1/1
  Demux2/1 -> Integrator4/1
  Demux2/2 -> Integrator5/1
  In1/1 -> Demux2/1
  Transfer Fcn1/1 -> Out2/1

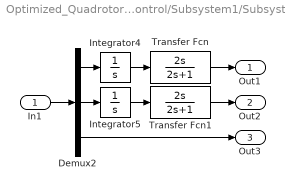
== system Optimized_Quadrotor_Trajectory_PID_Control/Subsystem1/Subsystem1 ==
  In1 : Inport
  Demux2 : Demux  Outputs=3
  Integrator4 : Integrator
  Integrator5 : Integrator
  Transfer Fcn : TransferFcn  Numerator=[2 0]  Denominator=[2 1]
  Transfer Fcn1 : TransferFcn  Numerator=[2 0]  Denominator=[2 1]
  Out1 : Outport  VectorParamsAs1DForOutWhenUnconnected=off
  Out2 : Outport  Port=2  VectorParamsAs1DForOutWhenUnconnected=off
  Out3 : Outport  Port=3  VectorParamsAs1DForOutWhenUnconnected=off
  wires:
  Transfer Fcn/1 -> Out1/1
  Integrator4/1 -> Transfer Fcn/1
  Integrator5/1 -> Transfer Fcn1/1
  Demux2/3 -> Out3/1
  Demux2/1 -> Integrator4/1
  Demux2/2 -> Integrator5/1
  In1/1 -> Demux2/1
  Transfer Fcn1/1 -> Out2/1

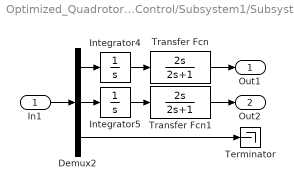
== system Optimized_Quadrotor_Trajectory_PID_Control/Subsystem1/Subsystem2 ==
  In1 : Inport
  Demux2 : Demux  Outputs=3
  Integrator4 : Integrator
  Integrator5 : Integrator
  Terminator : Terminator
  Transfer Fcn : TransferFcn  Numerator=[2 0]  Denominator=[2 1]
  Transfer Fcn1 : TransferFcn  Numerator=[2 0]  Denominator=[2 1]
  Out1 : Outport  VectorParamsAs1DForOutWhenUnconnected=off
  Out2 : Outport  Port=2  VectorParamsAs1DForOutWhenUnconnected=off
  wires:
  Transfer Fcn1/1 -> Out2/1
  In1/1 -> Demux2/1
  Demux2/2 -> Integrator5/1
  Demux2/1 -> Integrator4/1
  Demux2/3 -> Terminator/1
  Integrator5/1 -> Transfer Fcn1/1
  Integrator4/1 -> Transfer Fcn/1
  Transfer Fcn/1 -> Out1/1

== system Optimized_Quadrotor_Trajectory_PID_Control/Subsystem1/Derivative/Subsystem ==
  In1 : Inport
  Constant : Constant  Value=0.25
  MATLAB Function3 : MATLAB Function  TreatAsAtomicUnit=on
  Memory : Memory
  Out1 : Outport  VectorParamsAs1DForOutWhenUnconnected=off
  wires:
  Memory/1 -> MATLAB Function3/3(y_prev)
  Constant/1 -> MATLAB Function3/2(threshold)
  MATLAB Function3/1(y) -> Memory/1, Out1/1
  In1/1 -> MATLAB Function3/1(u)

== system Optimized_Quadrotor_Trajectory_PID_Control/Subsystem1/Derivative1/Subsystem ==
  In1 : Inport
  Constant : Constant  Value=0.25
  MATLAB Function3 : MATLAB Function  TreatAsAtomicUnit=on
  Memory : Memory
  Out1 : Outport  VectorParamsAs1DForOutWhenUnconnected=off
  wires:
  Memory/1 -> MATLAB Function3/3(y_prev)
  Constant/1 -> MATLAB Function3/2(threshold)
  MATLAB Function3/1(y) -> Memory/1, Out1/1
  In1/1 -> MATLAB Function3/1(u)

== system Optimized_Quadrotor_Trajectory_PID_Control/Subsystem1/Derivative2/Subsystem ==
  In1 : Inport
  Constant : Constant  Value=0.25
  MATLAB Function3 : MATLAB Function  TreatAsAtomicUnit=on
  Memory : Memory
  Out1 : Outport  VectorParamsAs1DForOutWhenUnconnected=off
  wires:
  In1/1 -> MATLAB Function3/1(u)
  MATLAB Function3/1(y) -> Out1/1, Memory/1
  Constant/1 -> MATLAB Function3/2(threshold)
  Memory/1 -> MATLAB Function3/3(y_prev)

== matlab function Optimized_Quadrotor_Trajectory_PID_Control/Subsystem1/MATLAB Function2 ==
  data: V input; dxi output; Omega input; eta input; deta output
function [dxi,deta] = fcn(V,Omega,eta)

phi = eta(1);
tta = eta(2);
psi = eta(3);

R = [cos(psi)*cos(tta)  -sin(psi)*cos(phi)+cos(psi)*sin(tta)*sin(phi)   sin(psi)*sin(phi)+cos(psi)*cos(phi)*sin(tta)
     sin(psi)*cos(tta)   cos(psi)*cos(phi)+sin(phi)*sin(tta)*sin(psi)  -cos(psi)*sin(phi)+sin(tta)*sin(psi)*cos(phi)
     -sin(tta)           cos(tta)*sin(phi)                              cos(tta)*cos(phi)];
 
W = [1  sin(phi)*tan(tta)   cos(phi)*tan(tta)
     0  cos(phi)           -sin(phi)
     0  sin(phi)/cos(tta)   cos(phi)/cos(tta)];

dxi = R*V;
deta = W*Omega;

== matlab function Optimized_Quadrotor_Trajectory_PID_Control/Subsystem1/MATLAB Function5 ==
  data: V input; dxi output; Omega input; eta input; deta output
function [dxi,deta] = fcn(V,Omega,eta)

phi = eta(1);
tta = eta(2);
psi = eta(3);

R = [cos(psi)*cos(tta)  -sin(psi)*cos(phi)+cos(psi)*sin(tta)*sin(phi)   sin(psi)*sin(phi)+cos(psi)*cos(phi)*sin(tta)
     sin(psi)*cos(tta)   cos(psi)*cos(phi)+sin(phi)*sin(tta)*sin(psi)  -cos(psi)*sin(phi)+sin(tta)*sin(psi)*cos(phi)
     -sin(tta)           cos(tta)*sin(phi)                              cos(tta)*cos(phi)];
 
W = [1  sin(phi)*tan(tta)   cos(phi)*tan(tta)
     0  cos(phi)           -sin(phi)
     0  sin(phi)/cos(tta)   cos(phi)/cos(tta)];

dxi = R*V;
deta = W*Omega;

== matlab function Optimized_Quadrotor_Trajectory_PID_Control/Subsystem1/Derivative1/Subsystem/MATLAB Function3 ==
  data: u input; y output; threshold input; y_prev input
function y = fcn(u,threshold,y_prev)
if abs(u - y_prev) > threshold
    y = y_prev;
else
    y = u;
end

== matlab function Optimized_Quadrotor_Trajectory_PID_Control/Subsystem1/QBall 2 Model 3/MATLAB Function6 ==
  data: Fz input; Tau input; Omega input; eta input; ddp output; dOmega output
function [ddp,dOmega] = fcn(Fz,Tau,Omega,eta)

Parametros = [  % Manufacturer
   1.79
   0.03
   0.00
   0.00
   0.03
   0.00
   0.04];

% Parametros = [  % 14-Jun-2019_18-33-20 T1E1
%    1.829678147298636
%    0.010093518395732
%   -0.000587374456966
%    0.003051684795895
%    0.020934240830821
%    0.000179364005119
%    0.105471993294800];

% Parametros = [  % 14-Jun-2019_18-36-38 T1E2
%    1.818755164320559
%    0.015372527142417
%   -0.003406485346485
%    0.002083178012305
%    0.019512061907602
%   -0.000620131329515
%    0.111022013170028];

% Parametros = [  % 20-Jun-2019_09-03-15 T2E1
%    1.814045169635898
%    0.009638937954855
%    0.000236321278316
%   -0.000440168241711
%    0.016271439845061
%   -0.001384767379204
%    0.084705097036282];

% Parametros = [  % 20-Jun-2019_09-07-19 T2E2
%    1.816449038428290
%    0.013453840218778
%    0.002848965863275
%   -0.000914261709212
%    0.013755836350366
%   -0.000964489425951
%    0.091879162538837];

% Parametros = [  % 20-Jun-2019_09-28-11 T2E3
%    1.808642457560659
%    0.011646527138149
%    0.002508639181441
%   -0.000559939657039
%    0.022996229568014
%   -0.000675956378368
%    0.091082362761357];

% Parametros = [  % 03-Jul-2019_11-44-51 T3E1
%    1.778776027879048
%    0.015880402609160
%    0.000921132391568
%    0.002043873620352
%    0.010672144758772
%    0.002653429938916
%    0.091385789990198];

% Parametros = [  % 03-Jul-2019_11-48-21 T3E2
%    1.785869074384763
%    0.010552973622277
%   -0.000116219938120
%    0.001165427701030
%    0.015552279444504
%    0.003206150645022
%    0.098577562109087];

% Parametros = [  % 03-Jul-2019_11-57-23 T4E1
%    1.737611579857987
%    0.022499330829682
%   -0.000701639931302
%   -0.000274522399987
%    0.019053102352100
%    0.002501032319942
%    0.095393148394978];

% Parametros = [  % 03-Jul-2019_12-05-29 T4E2
%    1.753732724782751
%    0.019833420574395
%   -0.001838988010042
%    0.000664719548222
%    0.017802221622542
%    0.002855090149509
%    0.104254468680096];

 m = Parametros(1); %Masa del quadrotor [Kg]
 g = 9.81;  %Accel. Gravitacional [m/s^2]
 Tensor = Parametros(2:7);
ez = [0;0;1];


 I = [Tensor(1)  Tensor(2)  Tensor(3);
      Tensor(2)  Tensor(4)  Tensor(5);
      Tensor(3)  Tensor(5)  Tensor(6)];

phi = eta(1);
tta = eta(2);
psi = eta(3);

R = [cos(psi)*cos(tta)  cos(psi)*sin(tta)*sin(phi)-sin(psi)*cos(phi)  cos(psi)*cos(phi)*sin(tta)+sin(psi)*sin(phi)
     sin(psi)*cos(tta)  sin(phi)*sin(tta)*sin(psi)+cos(psi)*cos(phi)  sin(tta)*sin(psi)*cos(phi)-cos(psi)*sin(phi)
     -sin(tta)          cos(tta)*sin(phi)                            cos(tta)*cos(phi)];

SOmega = [0        -Omega(3)  Omega(2);
          Omega(3)  0        -Omega(1);
         -Omega(2)  Omega(1)  0];
     
% G = m*g*R'*ez;

ddp    = (R*ez*Fz - m*g*ez)/m;
dOmega = I\(Tau - SOmega*I*Omega);

== matlab function Optimized_Quadrotor_Trajectory_PID_Control/Subsystem1/MATLAB Function7 ==
  data: Omega input; eta input; deta output
function deta  = fcn(Omega,eta)

phi = eta(1);
tta = eta(2);

 
W = [1  sin(phi)*tan(tta)   cos(phi)*tan(tta)
     0  cos(phi)           -sin(phi)
     0  sin(phi)/cos(tta)   cos(phi)/cos(tta)];

deta = W*Omega;

== matlab function Optimized_Quadrotor_Trajectory_PID_Control/Subsystem1/QBall 2 Model 3/MATLAB Function8 ==
  data: Omega input; eta input; deta output
function deta  = fcn(Omega,eta)

phi = eta(1);
tta = eta(2);

 
W = [1  sin(phi)*tan(tta)   cos(phi)*tan(tta)
     0  cos(phi)           -sin(phi)
     0  sin(phi)/cos(tta)   cos(phi)/cos(tta)];

deta = W*Omega;

== matlab function Optimized_Quadrotor_Trajectory_PID_Control/Subsystem1/Derivative2/Subsystem/MATLAB Function3 ==
  data: u input; y output; threshold input; y_prev input
function y = fcn(u,threshold,y_prev)
if abs(u - y_prev) > threshold
    y = y_prev;
else
    y = u;
end

== matlab function Optimized_Quadrotor_Trajectory_PID_Control/Subsystem1/MATLAB Function6 ==
  data: Omega input; eta input; deta output
function deta  = fcn(Omega,eta)

phi = eta(1);
tta = eta(2);

W = [1  sin(phi)*tan(tta)   cos(phi)*tan(tta)
     0  cos(phi)           -sin(phi)
     0  sin(phi)/cos(tta)   cos(phi)/cos(tta)];

deta = W*Omega;

== matlab function Optimized_Quadrotor_Trajectory_PID_Control/MATLAB Function ==
  data: T input; pd output; dpd output; ddpd output; psid output; dpsid output; ddpsid output
function [pd,dpd,ddpd,psid,dpsid,ddpsid] = fcn(T)
%% Vector de coeficientes para las trayectorias

% Trayectoria Optimizada el 14 de junio de 2019 (Experimentos del 14 al 19 de junio de 2019)
% x = [-0.0429849265144648,-0.0763064841152198,-0.0749350695407278,-0.0886858443349295,0.282912324505342,-0.0708904272116119,-0.0307981787056877,-0.0689233759650411,-0.0193304964522428,0.189942478334584,-0.0647769258075388,-0.0339154626109122,0.135647966215894,0.0208712206969480,-0.0578267984943908,-0.365497023615890,-0.311402556823631,1.28958970488918,-0.228632644705764,-0.384057480116424,-0.0560914444968585,-0.0263637738153223,-0.0461014536524470,-0.0797167924701083,0.113198104592526,0.182296797855871,0.203181761809395,0.144948506029630,0.0950457500551074,-0.280737767971053,0.0278315575719202,0.111165109243301,0.214759075994425,-0.0645063044014119,-0.127282757241108,-0.0502420167388700,-0.0236677947052981,0.163748441057463,0.0114618090695651,-0.0879029906671403,-0.130395740089182,0.477174739691477,0.880509307805824,-0.0353455217184256];

% Trayectoria Optimizada el 19 de junio de 2019 (Experimentos del 20 de junio de 2019)
% x = [-0.0999567302387145	-0.0385860166141405	-0.0827864104380497	-0.0698100822949648	0.291139239585869	-0.0163168425331471	0.0417536559571321	-0.00793071794584340	0.0146743988783628	-0.0321804943565044	-0.0338190832871314	-0.103904378450279	0.222400853928357	-0.0738358661521082	-0.0108415260388385	0.195925339827942	0.170940099330484	-0.0585619366077467	-0.260029652591294	-0.0482738499593855	-0.0711929755375397	0.0290321450151349	0.0218366953374294	0.0249274137816420	-0.0304182111255590	0.211243716107258	0.0830110237056274	0.0954124898419873	0.141818545665924	-0.246155483126367	0.0832594467067037	0.0414416481957701	0.201953574353016	-0.145679388875716	-0.0378571821547879	0.113649999920615	-0.213979065775385	0.172389684993490	-0.0428174325689645	-0.00631823861150646	-0.0783834806165133	0.430954870476641	0.902615137102785	0.0830083579535073];

% Trayectorias Optimizadas el 03 de julio de 2019 (Experimentos del 03 de julio de 2019)
% x = [-0.0889597242885246,-0.0596905118129632,-0.00768587719493194,-0.0355133768006474,0.191849490097067,0.141355992945595,0.00561307305711299,0.0105285194377162,0.0499599791050573,-0.207457564545482,0.0141391281826968,0.0212729774643029,-0.0884585831766713,0.0715469847682089,-0.0185005072385374,0.0308416148343187,0.0674854930266666,0.237337934858680,-0.316162923141082,-0.0195021195785831,0.282680479657463,0.115873963911995,0.0852363272011954,0.0588898573501207,-0.201139363697120,0.205653070376522,0.109084960197098,0.0778755432667148,0.0657544352662102,-0.184093472312325,0.0657314641888558,0.274146324906185,-0.0189542127491616,-0.366413841082292,0.181698777680797,0.0161630262080945,0.0103029947149329,-0.122101942698478,0.0962041778798820,-0.0110559798176909,0.546735684941094,0.422992425409643,0.924763147949273,0.00390522382830915];
% 
x = [0.191404252939832,-0.0288599052305868,0.0782465779202838,0.0111540925124213,-0.251945018141950,0.137500440031730,-0.0289063326725940,-0.0104599685760643,0.0213714541018399,-0.119505592884912,0.0151510395926445,0.0750495155139243,0.107341748585174,-0.439245154810725,0.241702851118983,-0.0429896587147428,-0.0682574267666725,-0.211588730557549,0.336857914515913,-0.0140220984769484,0.207912385030823,0.0805928667549614,0.0188483211351123,0.0223368527259053,-0.102998098565883,-0.229987649867433,-0.127183662237896,-0.100106054644828,-0.0978703210161752,0.235230884501957,0.105734791583532,0.177010705976995,0.125470501735700,-0.415241431814159,0.164959603686450,-0.0215259471482453,-0.0285208753584112,0.0934856604306096,-0.00644919278176279,-0.0352185024606928,0.381138186853304,-0.484419214673846,0.962995916654682,-0.0211365669734246];


%%
wf = 0.1*2*pi; % Frecuencia fundamental de la trayectoria
% Coeficientes de la serie de Fourier (5 armonicos)
ax   = x(1:5);
ay   = x(6:10);
az   = x(11:15);
apsi = x(16:20);
bx   = x(21:25);
by   = x(26:30);
bz   = x(31:35);
bpsi = x(36:40);
cx   = x(41);
cy   = x(42);
cz   = x(43);
cpsi = x(44);
%%

if T < 0

   xd       = 0;
   dxd      = 0;
   ddxd     = 0;
   
   yd       = 0;
   dyd      = 0;
   ddyd     = 0;
   
   zd       = 0.3;
   dzd      = 0;
   ddzd     = 0;
   
   psid     = 0;
   dpsid    = 0;
   ddpsid   = 0;

elseif T>=0 && T<=60
    % Vector de Trayectorias deseadas iniciales
xd      = cx;
yd      = cy;
zd      = cz;
psid    = cpsi;
dxd     = 0;
dyd     = 0;
dzd     = 0;
dpsid   = 0;
ddxd    = 0;
ddyd    = 0;
ddzd    = 0;
ddpsid  = 0;
for i = 1:5
   xd       = xd + ((ax(i)*sin(i*wf*T) - bx(i)*cos(i*wf*T))/(i*wf));
   dxd      = dxd + ax(i)*cos(i*wf*T) + bx(i)*sin(i*wf*T);
   ddxd     = ddxd + (i*wf)*(-ax(i)*sin(i*wf*T) + bx(i)*cos(i*wf*T));
   
   yd       = yd + ((ay(i)*sin(i*wf*T) - by(i)*cos(i*wf*T))/(i*wf));
   dyd      = dyd + ay(i)*cos(i*wf*T) + by(i)*sin(i*wf*T);
   ddyd     = ddyd + (i*wf)*(-ay(i)*sin(i*wf*T) + by(i)*cos(i*wf*T));
   
   zd       = zd + ((az(i)*sin(i*wf*T) - bz(i)*cos(i*wf*T))/(i*wf));
   dzd      = dzd + az(i)*cos(i*wf*T) + bz(i)*sin(i*wf*T);
   ddzd     = ddzd + (i*wf)*(-az(i)*sin(i*wf*T) + bz(i)*cos(i*wf*T));
   
   psid     = psid + ((apsi(i)*sin(i*wf*T) - bpsi(i)*cos(i*wf*T))/(i*wf));
   dpsid    = dpsid + apsi(i)*cos(i*wf*T) + bpsi(i)*sin(i*wf*T);
   ddpsid   = ddpsid + (i*wf)*(-apsi(i)*sin(i*wf*T) + bpsi(i)*cos(i*wf*T));
end
else
   xd       = 0;
   dxd      = 0;
   ddxd     = 0;
   
   yd       = 0;
   dyd      = 0;
   ddyd     = 0;
   
   zd       = 0.3;
   dzd      = 0;
   ddzd     = 0;
   
   psid     = 0;
   dpsid    = 0;
   ddpsid   = 0;
end
pd = [xd;yd;zd];
dpd = [dxd;dyd;dzd];
ddpd = [ddxd;ddyd;ddzd];

== matlab function Optimized_Quadrotor_Trajectory_PID_Control/Movement/MATLAB Function ==
  data: phi input; RT output; tta input; psi input
function RT = fcn(phi,tta,psi)

RT = [cos(tta)*cos(psi);
    sin(tta)*cos(psi)*sin(phi)-sin(psi)*cos(phi);
    sin(tta)*cos(psi)*cos(phi)+sin(psi)*sin(phi);
    cos(tta)*sin(psi);
    sin(tta)*sin(psi)*sin(phi)+cos(psi)*cos(phi);
    sin(tta)*sin(psi)*cos(phi)-cos(psi)*sin(phi);
    -sin(tta);
    cos(tta)*sin(phi);
    cos(tta)*cos(phi)];

== matlab function Optimized_Quadrotor_Trajectory_PID_Control/Subsystem1/MATLAB Function4 ==
  data: Fz input; Tau input; V input; Omega input; eta input; dV output; dOmega output
function [dV,dOmega] = fcn(Fz,Tau,V,Omega,eta)

Parametros = [  % Manufacturer
   1.79
   0.03
   0.00
   0.00
   0.03
   0.00
   0.04];

% Parametros = [  % 14-Jun-2019_18-33-20 T1E1
%    1.829678147298636
%    0.010093518395732
%   -0.000587374456966
%    0.003051684795895
%    0.020934240830821
%    0.000179364005119
%    0.105471993294800];

% Parametros = [  % 14-Jun-2019_18-36-38 T1E2
%    1.818755164320559
%    0.015372527142417
%   -0.003406485346485
%    0.002083178012305
%    0.019512061907602
%   -0.000620131329515
%    0.111022013170028];

% Parametros = [  % 20-Jun-2019_09-03-15 T2E1
%    1.814045169635898
%    0.009638937954855
%    0.000236321278316
%   -0.000440168241711
%    0.016271439845061
%   -0.001384767379204
%    0.084705097036282];

% Parametros = [  % 20-Jun-2019_09-07-19 T2E2
%    1.816449038428290
%    0.013453840218778
%    0.002848965863275
%   -0.000914261709212
%    0.013755836350366
%   -0.000964489425951
%    0.091879162538837];

% Parametros = [  % 20-Jun-2019_09-28-11 T2E3
%    1.808642457560659
%    0.011646527138149
%    0.002508639181441
%   -0.000559939657039
%    0.022996229568014
%   -0.000675956378368
%    0.091082362761357];

% Parametros = [  % 03-Jul-2019_11-44-51 T3E1
%    1.778776027879048
%    0.015880402609160
%    0.000921132391568
%    0.002043873620352
%    0.010672144758772
%    0.002653429938916
%    0.091385789990198];

% Parametros = [  % 03-Jul-2019_11-48-21 T3E2
%    1.785869074384763
%    0.010552973622277
%   -0.000116219938120
%    0.001165427701030
%    0.015552279444504
%    0.003206150645022
%    0.098577562109087];

% Parametros = [  % 03-Jul-2019_11-57-23 T4E1
%    1.737611579857987
%    0.022499330829682
%   -0.000701639931302
%   -0.000274522399987
%    0.019053102352100
%    0.002501032319942
%    0.095393148394978];

% Parametros = [  % 03-Jul-2019_12-05-29 T4E2
%    1.753732724782751
%    0.019833420574395
%   -0.001838988010042
%    0.000664719548222
%    0.017802221622542
%    0.002855090149509
%    0.104254468680096];

 m = Parametros(1); %Masa del quadrotor [Kg]
 g = 9.81;  %Accel. Gravitacional [m/s^2]
 Tensor = Parametros(2:7);
ez = [0;0;1];


 I = [Tensor(1)  Tensor(2)  Tensor(3);
      Tensor(2)  Tensor(4)  Tensor(5);
      Tensor(3)  Tensor(5)  Tensor(6)];

phi = eta(1);
tta = eta(2);
psi = eta(3);

R = [cos(psi)*cos(tta)  cos(psi)*sin(tta)*sin(phi)-sin(psi)*cos(phi)  cos(psi)*cos(phi)*sin(tta)+sin(psi)*sin(phi)
     sin(psi)*cos(tta)  sin(phi)*sin(tta)*sin(psi)+cos(psi)*cos(phi)  sin(tta)*sin(psi)*cos(phi)-cos(psi)*sin(phi)
     -sin(tta)          cos(tta)*sin(phi)                            cos(tta)*cos(phi)];

SOmega = [0        -Omega(3)  Omega(2);
          Omega(3)  0        -Omega(1);
         -Omega(2)  Omega(1)  0];
     
G = m*g*R'*ez;

dV     = (Fz*ez - m*SOmega*V - G)/m;
dOmega = I\(Tau - SOmega*I*Omega);

== matlab function Optimized_Quadrotor_Trajectory_PID_Control/Subsystem1/Derivative/Subsystem/MATLAB Function3 ==
  data: u input; y output; threshold input; y_prev input
function y = fcn(u,threshold,y_prev)
if abs(u - y_prev) > threshold
    y = y_prev;
else
    y = u;
end

== matlab function Optimized_Quadrotor_Trajectory_PID_Control/PID Controller/Orientation/Orientation Controller ==
  data: en input; eta input; den input; deta input; ien input; Tau output; ddetad input; detad input
function Tau  = fcn(en, eta, den, deta, ien, ddetad, detad)

I = [0.013832055669759   0.001591901145665  -0.000244508007647  % Parametros Identificados
     0.001591901145665   0.014564426773424  -0.000675767460689
    -0.000244508007647  -0.000675767460689   0.001348725526523];

kpphi = 2.0;
kptta = 2.0;
kppsi = 2.6;
Kp = [kpphi 0 0;0 kptta 0;0 0 kppsi];

kdphi = 0.6;
kdtta = 0.6;
kdpsi = 1.0;
Kd = [kdphi 0 0;0 kdtta 0;0 0 kdpsi];

kiphi = 0.03;
kitta = 0.05;
kipsi = 0.01;
Ki = [kiphi 0 0;0 kitta 0;0 0 kipsi];

phi = eta(1);
tta = eta(2);
 
W = [1  sin(phi)*tan(tta)   cos(phi)*tan(tta)
     0  cos(phi)           -sin(phi)
     0  sin(phi)/cos(tta)   cos(phi)/cos(tta)];
 
iW = [1 0         -sin(tta)
      0 cos(phi)  cos(tta)*sin(phi)
      0 -sin(phi) cos(tta)*cos(phi)];
  
dW = [0 cos(phi)*tan(tta)+sin(phi)*sec(tta)^2        -sin(phi)*tan(tta)+cos(phi*sec(tta)^2)
      0 -sin(phi)                                    -cos(phi)
      0 cos(phi)*sec(tta)+sin(phi)*sec(tta)*tan(tta) -sin(phi)*sec(tta)+cos(phi)*tan(tta)+cos(phi)*sec(tta)*tan(tta)];

iWdeta = iW*deta;

SiWdeta = [ 0         -iWdeta(3)  iWdeta(2)
            iWdeta(3)  0         -iWdeta(1)
           -iWdeta(2)  iWdeta(1)  0];

Ho = iW'*I*iW;
Co = iW'*(SiWdeta*I - I*iW*dW)*iW;

Tau = W'*(Kp*en + Ki*ien + Kd*den + Ho*ddetad + Co*detad);

== matlab function Optimized_Quadrotor_Trajectory_PID_Control/Subsystem1/MATLAB Function3 ==
  data: Omega input; eta input; deta output
function deta  = fcn(Omega,eta)

phi = eta(1);
tta = eta(2);
 
W = [1  sin(phi)*tan(tta)   cos(phi)*tan(tta)
     0  cos(phi)           -sin(phi)
     0  sin(phi)/cos(tta)   cos(phi)/cos(tta)];
 
deta = W*Omega;
